simulink library "Environment_Lib"  (Simulink 7.5)
settings: Solver=ode45  SolverMode=SingleTasking  StartTime=0.0  StopTime=10.0  RelTol=1e-3
values from neighbouring files (symbols this model uses):
  Env =     [UAV_modelconfig.mat]
undefined symbols (not defined in the file or in its folder): aeroassertmsg, F, Light, MIL
libraries: simulink x5, aerolibgravity2 x4, Environment_Lib x4, aerolibconvert2 x2, aerolibwind2 x2, aerolibatmos2 x1, aerolibutil x1
settings Model: Creator=Paul Freeman  LastModifiedBy=austinmurch

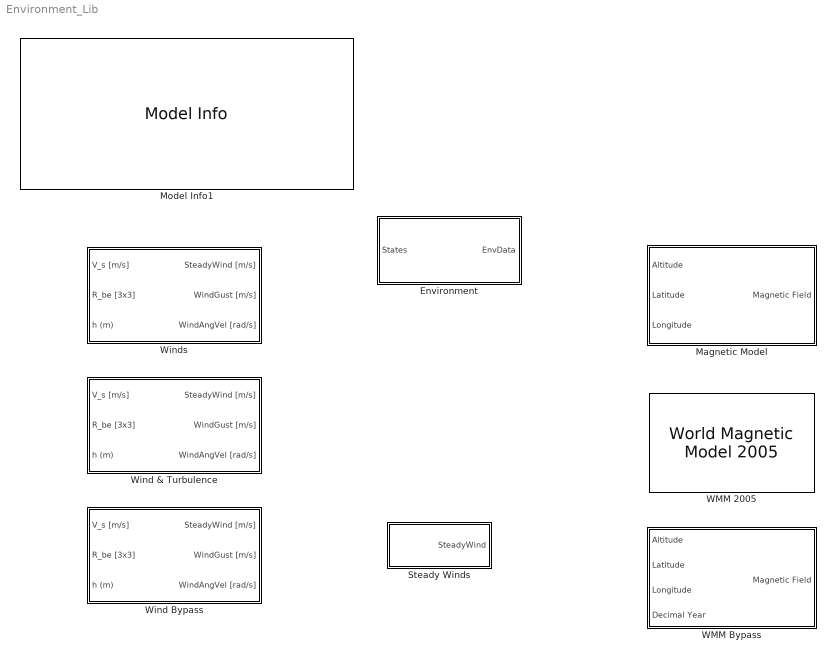
== system Environment_Lib ==
  Environment : Subsystem
  Magnetic Model : Subsystem  BlockChoice=WMM 2005
      settings: TemplateBlock=self  MemberBlocks=WMM 2005,WMM Bypass
  Model Info1 : simulink/Model-Wide Utilities/Model Info  SystemSampleTime=-1  InitialBlockCM=None  BlockCM=None  Frame=on  DisplayStringWithTags=|  HorizontalTextAlignment=Left  LeftAlignmentValue=0.02  SourceBlockDiagram=Environment_Lib  TagMaxNumber=20
      | MODEL INFORMATION
      | Environment Library
      | 
      | University of Minnesota
      | Aerospace Engineering and Mechanics
      | Copyright 2011 Regents of the University of Minnesota. All rights reserved.
      | 
      | == SVN Info ==
      | %<ModelVersion>
      | Last modified by %<LastModifiedBy> on %<LastModificationDate>
  Steady Winds : Subsystem
  WMM 2005 : aerolibgravity2/World Magnetic Model 2005  SystemSampleTime=-1  units=Metric (MKS)  time_in=on  month=August  day=1  year=2009  action=None  h_out=off  dec_out=off  inc_out=off  ti_out=off
  WMM Bypass : Subsystem  AncestorBlock=aerolibgravity2/World Magnetic Model 2005  mask(World Magnetic Model 2005){units=Metric (MKS), time_in=on, month=August, day=1, year=2009, action=None, h_out=off, dec_out=off, inc_out=off, ti_out=off}
      mask prompts: time_in "Input decimal year"; action "Action for out of range input:"; h_out "Output horizontal intensity"; dec_out "Output declination"; inc_out "Output inclination"; ti_out "Output total intensity"
      mask help:
      | Calculate the Earth's magnetic field at a specific location and time using the World Magnetic Model (WMM). This model is valid for the year 2005 through the year 2010.
      |
      | The WMM-2005 can be found on the web at http://www.ngdc.noaa.gov/seg/WMM/DoDWMM.shtml and in "NOAA Technical Report: The US/UK World Magnetic Model for 2005-2010 ".
      |
      | Height is entered in length units of selected unit system. Latitude and longitude are entered in degrees.
      mask init:
      | [ports,dyear,maxdef,epoch,c,cd,fn,fm,snorm,k]=aeroicon('aeroblkwmm2005','icon');
      mask Help: eval('asbhelp');
      mask StyleString: popup(Metric (MKS)|English),checkbox,popup(January|February|March|April|May|June|July|August|September|October|November|December),popup(1|2|3|4|5|6|7|8|9|10|11|12|13|14|15|16|17|18|19|20|21|22|23|24|25|26|27|28|29|30|31),popup(2005|2006|2007|2008|2009|2010),popup(None|Warning|Error),checkbox,checkbox,checkbox,checkbox
      mask CallbackString: |aeroicon('aeroblkwmm');|aeroicon('aeroblkwmm');|aeroicon('aeroblkwmm');|aeroicon('aeroblkwmm');|||||
      mask Display:
      | port_label(ports(1).type,ports(1).port,ports(1).txt);
      | port_label(ports(2).type,ports(2).port,ports(2).txt,'texmode','on');
      | port_label(ports(3).type,ports(3).port,ports(3).txt,'texmode','on');
      | port_label(ports(4).type,ports(4).port,ports(4).txt);
      | port_label(ports(5).type,ports(5).port,ports(5).txt);
      | port_label(ports(6).type,ports(6).port,ports(6).txt);
      | port_label(ports(7).type,ports(7).port,ports(7).txt);
      | port_label(ports(8).type,ports(8).port,ports(8).txt);
      | port_label(ports(9).type,ports(9).port,ports(9).txt);
  Wind & Turbulence : Subsystem
  Wind Bypass : Subsystem
      settings: MinAlgLoopOccurrences=on
  Winds : Subsystem  BlockChoice=Wind & Turbulence
      settings: TemplateBlock=self  MemberBlocks=Wind & Turbulence,Wind Bypass

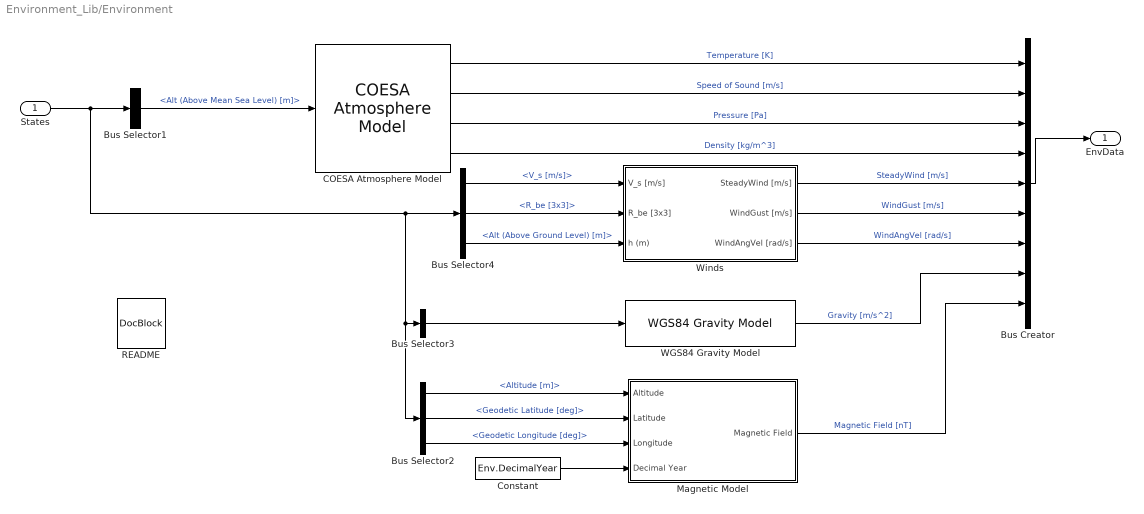
== system Environment_Lib/Environment ==
  States : Inport  OutDataType=sfix(16)  OutScaling=2^0
  Bus Creator : BusCreator  Inputs=9
  Bus Selector1 : BusSelector  OutputSignals=Nav.Alt (Above Mean Sea Level) [m]
  Bus Selector2 : BusSelector  OutputSignals=Nav.Altitude [m],Nav.Geodetic Latitude [deg],Nav.Geodetic Longitude [deg]
  Bus Selector3 : BusSelector  OutputSignals=Nav.Geodetic Latitude [deg],Nav.Geodetic Longitude [deg],Nav.Altitude [m]  OutputAsBus=on
  Bus Selector4 : BusSelector  OutputSignals=WindAxesParam.V_s [m/s],R_be [3x3],Nav.Alt (Above Ground Level) [m]
  COESA Atmosphere Model : aerolibatmos2/COESA Atmosphere Model  SystemSampleTime=-1  units=Metric (MKS)  spec=1976 COESA-extended U.S. Standard Atmosphere  model=Profile  profile_var=High temperature  profile_percent=1%  profile_alt=5 km (16404 ft)  envelope_var=High temperature  envelope_percent=1%  action=Warning
  Constant : Constant  Value=Env.DecimalYear  OutDataType=fixdt(1, 16)  OutScaling=2^0
  Magnetic Model : Subsystem  BlockChoice=WMM 2005
      settings: AttributesFormatString=%<BlockChoice>  TemplateBlock=Environment_Lib/Magnetic Model  MemberBlocks=WMM 2005,WMM Bypass
  README : simulink/Model-Wide Utilities/DocBlock  SystemSampleTime=-1  DocumentType=Text
      content=|
      | Environment Model
      |
      | This block uses the Aerospace Blockset models for Earth's atmosphere,
      | gravity, magnetic field, and wind.
      |
      | The atmosphere is modeled using the 1976 Standard Atmosphere block.
      |
      | Winds are modeled in two portions: steady and unsteady. The steady
      | portion is defined by a speed and direction, and is horizontal only. The
      | unsteady portion is made up of a wind gust model and a turbulence model.
      |
      | The Dryden Wind Turbulence Model is used to model turbulence. The
      | intensity of the turbulence at low altitude (<1000ft) is determined by
      | the wind speed and direction; this is set as separate variables from the
      | steady wind speed and direction. The turbulence is off by default, and
      | can be enabled by setting the Env.Winds.TurbulenceOn boolean in
      | UAV_config.m.
      |
      | The Discrete Gust Model is used to model wind gusts. Parameters are time
      | on, duration (length), and amplitude, in three axes (u,v,w). These
      | parameters are set in Env.Winds, in UAV_config.m
      |
      | Note the booleans in the Env.Winds stucture to turn on each wind
      | component: >> Env.Winds
      |
      | ans =
      |
      |      TurbulenceOn: 0
      |     TurbWindSpeed: 0
      |       TurbWindDir: 0
      |            GustOn: 0
      |     GustStartTime: 0
      |        GustLength: [1 1 1]
      |     GustAmplitude: [1 1 1]
      |      SteadyWindOn: 0
      |         WindSpeed: 0
      |           WindDir: 0
      |
      |
      | The WGS84 Gravity Model is used to model Earth's gravity as a function of
      | latitude, longitude, and altitude.
      |
      | The World Magnetic Model 2005 is used to model Earth's magnetic field as
      | a function of latitude, longitude, and altitude. The current decimal year
      | is input.
      |
      | *Note for trim/linearizing: the Dryden turbulence model and the World
      | Magnetic Model 2005 have many internal states, which makes trimming and
      | linearizing difficult. Thus "Bypass" blocks are substituted for the Winds
      | and Magnetic Model blocks using Configurable Subsystems. For the
      | UAV_NL.mdl, the block choices are automatically set to "Bypass" using the
      | models "InitFcn" callback, which can be viewed by using the Model
      | Explorer, selecting UAV_NL, and going to the "Callbacks" tab. The Nonlinear
      | UAV Model block will then show up as a Parameterized Link (red arrow in the
      | lower left corner). The SIL and PIL sims use the default blocks, and should
      | have a normal library link (black arrow).
  "WGS84 Gravity Model " : aerolibgravity2/WGS84 Gravity Model   SystemSampleTime=-1  model=WGS84 Taylor Series  units=Metric (MKS)  no_atmos=on  precessing=on  jd_loc=off  month=October  day=10  year=2004  no_centrifugal=on  action=Warning
  Winds : Subsystem  BlockChoice=Wind & Turbulence
      settings: AttributesFormatString=%<BlockChoice>  TemplateBlock=Environment_Lib/Winds  MemberBlocks=Wind & Turbulence,Wind Bypass
  EnvData : Outport  OutDataType=sfix(16)  OutScaling=2^0
  wires:
  Bus Selector4/3 -> Winds/3(h (m))  "<Alt (Above Ground Level) [m]>"
  Bus Selector4/2 -> Winds/2(R_be [3x3])  "<R_be [3x3]>"
  Bus Selector4/1 -> Winds/1(V_s [m/s])  "<V_s [m/s]>"
  Bus Creator/1 -> EnvData/1
  Bus Selector1/1 -> COESA Atmosphere Model/1  "<Alt (Above Mean Sea Level) [m]>"
  States/1 -> Bus Selector4/1, Bus Selector3/1, Bus Selector2/1, Bus Selector1/1
  COESA Atmosphere Model/3 -> Bus Creator/3  "Pressure [Pa]"
  COESA Atmosphere Model/2 -> Bus Creator/2  "Speed of Sound [m/s]"
  COESA Atmosphere Model/1 -> Bus Creator/1  "Temperature [K]"
  COESA Atmosphere Model/4 -> Bus Creator/4  "Density [kg/m^3]"
  Winds/1(SteadyWind [m/s]) -> Bus Creator/5  "SteadyWind [m/s]"
  Winds/2(WindGust [m/s]) -> Bus Creator/6  "WindGust [m/s]"
  Winds/3(WindAngVel [rad/s]) -> Bus Creator/7  "WindAngVel [rad/s]"
  "WGS84 Gravity Model "/1 -> Bus Creator/8  "Gravity [m/s^2]"
  Magnetic Model/1(Magnetic Field) -> Bus Creator/9  "Magnetic Field [nT]"
  Bus Selector2/1 -> Magnetic Model/1(Altitude)  "<Altitude [m]>"
  Bus Selector2/2 -> Magnetic Model/2(Latitude)  "<Geodetic Latitude [deg]>"
  Bus Selector2/3 -> Magnetic Model/3(Longitude)  "<Geodetic Longitude [deg]>"
  Bus Selector3/1 -> "WGS84 Gravity Model "/1
  Constant/1 -> Magnetic Model/4(Decimal Year)

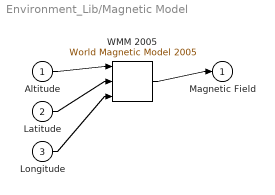
== system Environment_Lib/Magnetic Model ==
  Altitude : Inport
  Latitude : Inport  Port=2
  Longitude : Inport  Port=3
  WMM 2005 : aerolibgravity2/World Magnetic Model 2005  SystemSampleTime=-1  units=Metric (MKS)  time_in=off  month=August  day=1  year=2009  action=None  h_out=off  dec_out=off  inc_out=off  ti_out=off
  Magnetic Field : Outport
  wires:
  Altitude/1 -> WMM 2005/1
  Latitude/1 -> WMM 2005/2
  Longitude/1 -> WMM 2005/3
  WMM 2005/1 -> Magnetic Field/1

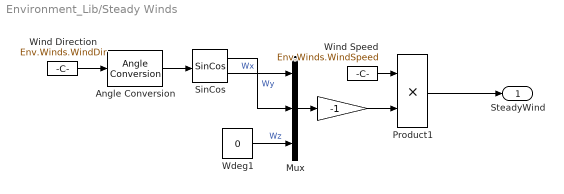
== system Environment_Lib/Steady Winds ==
  " " : Gain  Gain=-1  ParameterDataType=sfix(16)  ParameterScaling=2^0  OutDataType=sfix(16)  OutScaling=2^0  SaturateOnIntegerOverflow=on  OutDataTypeStr=Inherit: Same as input  ParamDataTypeStr=Inherit: Same as input
  Angle Conversion : aerolibconvert2/Angle Conversion  SystemSampleTime=-1  IU=deg  OU=rad
  Mux : Mux  Inputs=3
  Product1 : Product  OutDataType=sfix(16)  OutScaling=2^0  SaturateOnIntegerOverflow=on  InputSameDT=on  OutDataTypeStr=Inherit: Same as first input
  SinCos : aerolibutil/SinCos  SystemSampleTime=-1
  Wdeg1 : Constant  Value=0  OutDataType=sfix(16)  OutScaling=2^0  OutDataTypeStr=Inherit: Inherit via back propagation
  Wind Direction : Constant  Value=Env.Winds.WindDir  OutDataType=sfix(16)  OutScaling=2^0  OutDataTypeStr=Inherit: Inherit via back propagation
  Wind Speed : Constant  Value=Env.Winds.WindSpeed  OutDataType=sfix(16)  OutScaling=2^0  OutDataTypeStr=Inherit: Inherit via back propagation
  SteadyWind : Outport  OutDataType=fixdt(1, 16)  OutScaling=2^0
  wires:
  " "/1 -> Product1/2
  Product1/1 -> SteadyWind/1
  Mux/1 -> " "/1
  Wdeg1/1 -> Mux/3  "Wz"
  Angle Conversion/1 -> SinCos/1
  SinCos/1 -> Mux/2  "Wy"
  SinCos/2 -> Mux/1  "Wx"
  Wind Speed/1 -> Product1/1
  Wind Direction/1 -> Angle Conversion/1

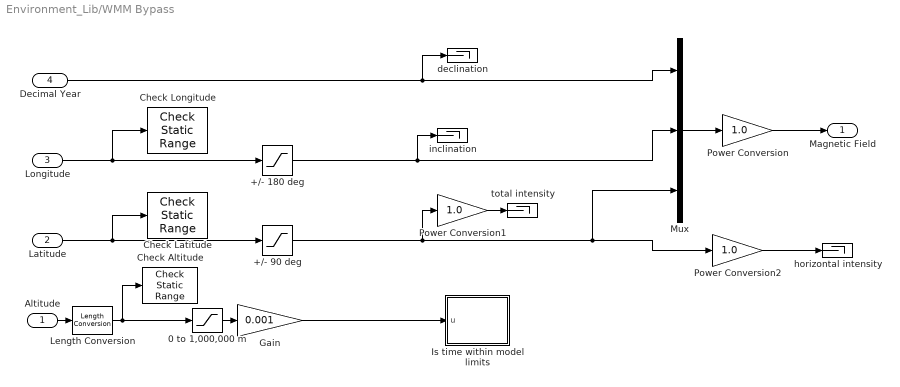
== system Environment_Lib/WMM Bypass ==
  Altitude : Inport  OutDataType=sfix(16)  OutScaling=2^0
  Latitude : Inport  Port=2  OutDataType=sfix(16)  OutScaling=2^0
  Longitude : Inport  Port=3  OutDataType=sfix(16)  OutScaling=2^0
  Decimal Year : Inport  Port=4
  +/- 180 deg : Saturate  UpperLimit=180.0  LowerLimit=-180.0  OutDataType=sfix(16)  OutScaling=2^0
  +/- 90 deg : Saturate  UpperLimit=90.0  LowerLimit=-90.0  OutDataType=sfix(16)  OutScaling=2^0
  0 to 1,000,000 m : Saturate  UpperLimit=1000000.0  LowerLimit=0  OutDataType=sfix(16)  OutScaling=2^0
  Check Altitude : simulink/Model Verification/Check  Static Range  Description=0 <= u <= 1000000  SystemSampleTime=-1  max=1000000  max_included=on  min=0  min_included=on  enabled=off  callback=aeroassertmsg('aeroblkwmm','alt');  stopWhenAssertionFail=off  export=off  icon=graphic
  Check Latitude : simulink/Model Verification/Check  Static Range  Description=-90 <= u <= 90  SystemSampleTime=-1  max=90  max_included=on  min=-90  min_included=on  enabled=off  callback=aeroassertmsg('aeroblkwmm','lat');  stopWhenAssertionFail=off  export=off  icon=graphic
  Check Longitude : simulink/Model Verification/Check  Static Range  Description=-180 <= u <= 180  SystemSampleTime=-1  max=180  max_included=on  min=-180  min_included=on  enabled=off  callback=aeroassertmsg('aeroblkwmm','lon');  stopWhenAssertionFail=off  export=off  icon=graphic
  Gain : Gain  Gain=0.001  ParameterDataType=sfix(16)  ParameterScaling=2^0  OutDataType=sfix(16)  OutScaling=2^0  SaturateOnIntegerOverflow=on  OutDataTypeStr=Inherit: Same as input  ParamDataTypeStr=Inherit: Same as input
  Is time within model limits : Subsystem  Description=0 <= u <= 5  mask(Checks_SRange){max=5, max_included=on, min=0, min_included=on, enabled=off, callback=aeroassertmsg('aeroblkwmm','time');, stopWhenAssertionFail=off, export=off, icon=graphic}
      mask prompts: max "Upper bound:"; max_included "Inclusive upper bound"; min "Lower bound:"; min_included "Inclusive lower bound"; enabled "Enable assertion"; callback "Simulation callback when assertion fails (optional):"; stopWhenAssertionFail "Stop simulation when assertion fails"; export "Output assertion signal"; icon "Select icon type:"
      mask help: Assert that the input signal lies between a static lower and upper bound or optionally equals either bound.
      mask init:
      | update_assert_sys(gcbh);
      mask StyleString: edit,checkbox,edit,checkbox,checkbox,edit,checkbox,checkbox,popup(graphic|text)
      mask Display:
      | image(imread('Checks_SRange.bmp','bmp'),'center')
      | plot([0 1], [0 1]);
      | plot([0 1],[1 0]);
  Length Conversion : aerolibconvert2/Length Conversion  SystemSampleTime=-1  IU=m  OU=m
  Mux : Mux  Inputs=3
  Power Conversion : Gain  Gain=1.0  ParameterDataType=sfix(16)  ParameterScaling=2^0  OutDataType=sfix(16)  OutScaling=2^0  SaturateOnIntegerOverflow=on  OutDataTypeStr=Inherit: Same as input  ParamDataTypeStr=Inherit: Same as input
  Power Conversion1 : Gain  Gain=1.0  ParameterDataType=sfix(16)  ParameterScaling=2^0  OutDataType=sfix(16)  OutScaling=2^0  SaturateOnIntegerOverflow=on  OutDataTypeStr=Inherit: Same as input  ParamDataTypeStr=Inherit: Same as input
  Power Conversion2 : Gain  Gain=1.0  ParameterDataType=sfix(16)  ParameterScaling=2^0  OutDataType=sfix(16)  OutScaling=2^0  SaturateOnIntegerOverflow=on  OutDataTypeStr=Inherit: Same as input  ParamDataTypeStr=Inherit: Same as input
  declination : Terminator
  horizontal intensity : Terminator
  inclination : Terminator
  total intensity : Terminator
  Magnetic Field : Outport  OutDataType=sfix(16)  OutScaling=2^0
  wires:
  Altitude/1 -> Length Conversion/1
  Length Conversion/1 -> 0 to 1,000,000 m/1, Check Altitude/1
  Decimal Year/1 -> declination/1, Mux/1
  Latitude/1 -> +/- 90 deg/1, Check Latitude/1
  Longitude/1 -> +/- 180 deg/1, Check Longitude/1
  Gain/1 -> Is time within model limits/1(u)
  Mux/1 -> Power Conversion/1
  Power Conversion/1 -> Magnetic Field/1
  Power Conversion1/1 -> total intensity/1
  Power Conversion2/1 -> horizontal intensity/1
  +/- 90 deg/1 -> Power Conversion1/1, Power Conversion2/1, Mux/3
  +/- 180 deg/1 -> inclination/1, Mux/2
  0 to 1,000,000 m/1 -> Gain/1

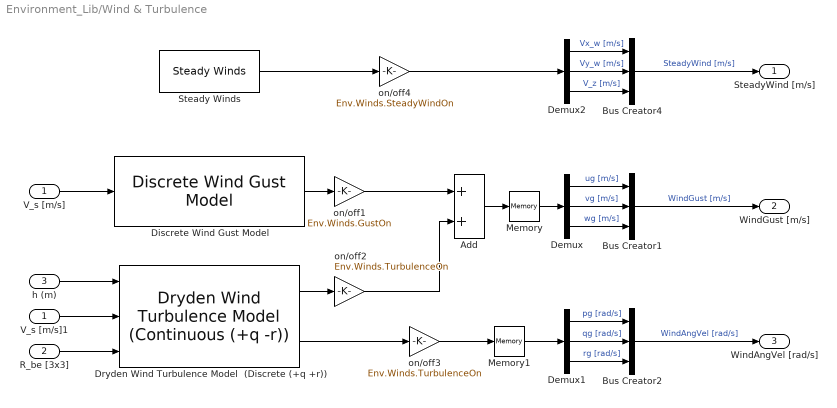
== system Environment_Lib/Wind & Turbulence ==
  V_s [m/s] : Inport  OutDataType=sfix(16)  OutScaling=2^0
  R_be [3x3] : Inport  Port=2  OutDataType=sfix(16)  OutScaling=2^0
  h (m) : Inport  Port=3  OutDataType=sfix(16)  OutScaling=2^0
  Add : Sum  OutDataType=fixdt(1, 16)  OutScaling=2^-10
  Bus Creator1 : BusCreator  Inputs=3
  Bus Creator2 : BusCreator  Inputs=3
  Bus Creator4 : BusCreator  Inputs=3
  Demux : Demux  Outputs=3
  Demux1 : Demux  Outputs=3
  Demux2 : Demux  Outputs=3
  Discrete Wind Gust Model : aerolibwind2/Discrete Wind Gust Model  SystemSampleTime=-1  units=Metric (MKS)  Gx=on  Gy=on  Gz=on  t_0=Env.Winds.GustStartTime  d_m=Env.Winds.GustLength  v_m=Env.Winds.GustAmplitude
  Dryden Wind Turbulence Model  (Discrete (+q +r)) : aerolibwind2/Dryden Wind Turbulence Model  (Continuous (+q -r))  SystemSampleTime=-1  units=Metric (MKS)  spec=MIL-F-8785C  model=Discrete Dryden (+q +r)  W20=Env.Winds.TurbWindSpeed  Wdeg=Env.Winds.TurbWindDir  TurbProb=10^-2 - Light  L_high=762  Wingspan=AC.Geometry.b  ts=SampleTime  Seed=[23341 23342 23343 23344]  T_on=on
  Memory : Memory
  Memory1 : Memory
  Steady Winds : Environment_Lib/Steady Winds  SystemSampleTime=-1
  V_s [m/s]1 : InportShadow  Port=1  OutDataType=sfix(16)  OutScaling=2^0
  on/off1 : Gain  Gain=Env.Winds.GustOn  ParameterDataType=fixdt(1, 16)  ParameterScaling=2^0  OutDataType=fixdt(1, 16)  OutScaling=2^0
  on/off2 : Gain  Gain=Env.Winds.TurbulenceOn  ParameterDataType=fixdt(1, 16)  ParameterScaling=2^0  OutDataType=fixdt(1, 16)  OutScaling=2^0
  on/off3 : Gain  Gain=Env.Winds.TurbulenceOn  ParameterDataType=fixdt(1, 16)  ParameterScaling=2^0  OutDataType=fixdt(1, 16)  OutScaling=2^0
  on/off4 : Gain  Gain=Env.Winds.SteadyWindOn  ParameterDataType=fixdt(1, 16)  ParameterScaling=2^0  OutDataType=fixdt(1, 16)  OutScaling=2^0
  SteadyWind [m/s] : Outport  OutDataType=sfix(16)  OutScaling=2^0
  WindGust [m/s] : Outport  Port=2  OutDataType=sfix(16)  OutScaling=2^0
  WindAngVel [rad/s] : Outport  Port=3  OutDataType=sfix(16)  OutScaling=2^0
  wires:
  Demux/1 -> Bus Creator1/1  "ug [m/s]"
  Demux1/3 -> Bus Creator2/3  "rg [rad/s]"
  Demux1/2 -> Bus Creator2/2  "qg [rad/s]"
  Demux1/1 -> Bus Creator2/1  "pg [rad/s]"
  Demux/3 -> Bus Creator1/3  "wg [m/s]"
  Demux/2 -> Bus Creator1/2  "vg [m/s]"
  V_s [m/s]/1 -> Discrete Wind Gust Model/1
  Demux2/1 -> Bus Creator4/1  "Vx_w [m/s]"
  Demux2/3 -> Bus Creator4/3  "V_z [m/s]"
  Demux2/2 -> Bus Creator4/2  "Vy_w [m/s]"
  Steady Winds/1 -> on/off4/1
  Add/1 -> Memory/1
  Discrete Wind Gust Model/1 -> on/off1/1
  Dryden Wind Turbulence Model  (Discrete (+q +r))/1 -> on/off2/1
  on/off3/1 -> Memory1/1
  on/off4/1 -> Demux2/1
  on/off1/1 -> Add/1
  on/off2/1 -> Add/2
  Memory/1 -> Demux/1
  Memory1/1 -> Demux1/1
  Bus Creator4/1 -> SteadyWind [m/s]/1  "SteadyWind [m/s]"
  Bus Creator1/1 -> WindGust [m/s]/1  "WindGust [m/s]"
  Bus Creator2/1 -> WindAngVel [rad/s]/1  "WindAngVel [rad/s]"
  Dryden Wind Turbulence Model  (Discrete (+q +r))/2 -> on/off3/1
  R_be [3x3]/1 -> Dryden Wind Turbulence Model  (Discrete (+q +r))/3
  h (m)/1 -> Dryden Wind Turbulence Model  (Discrete (+q +r))/1
  V_s [m/s]1/1 -> Dryden Wind Turbulence Model  (Discrete (+q +r))/2

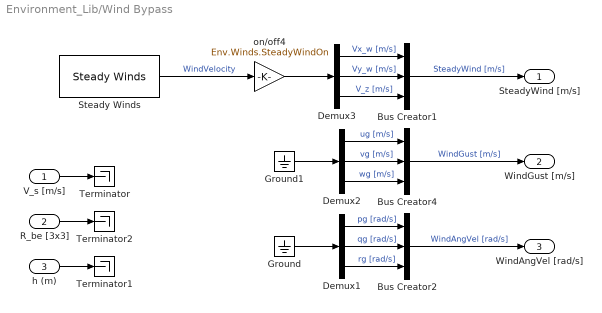
== system Environment_Lib/Wind Bypass ==
  V_s [m/s] : Inport  OutDataType=sfix(16)  OutScaling=2^0
  R_be [3x3] : Inport  Port=2  OutDataType=sfix(16)  OutScaling=2^0
  h (m) : Inport  Port=3  OutDataType=sfix(16)  OutScaling=2^0
  Bus Creator1 : BusCreator  Inputs=3
  Bus Creator2 : BusCreator  Inputs=3
  Bus Creator4 : BusCreator  Inputs=3
  Demux1 : Demux  Outputs=3
  Demux2 : Demux  Outputs=3
  Demux3 : Demux  Outputs=3
  Ground : Ground
  Ground1 : Ground
  Steady Winds : Environment_Lib/Steady Winds  SystemSampleTime=-1
  Terminator : Terminator
  Terminator1 : Terminator
  Terminator2 : Terminator
  on/off4 : Gain  Gain=Env.Winds.SteadyWindOn  ParameterDataType=fixdt(1, 16)  ParameterScaling=2^0  OutDataType=fixdt(1, 16)  OutScaling=2^0
  SteadyWind [m/s] : Outport  OutDataType=sfix(16)  OutScaling=2^0
  WindGust [m/s] : Outport  Port=2  OutDataType=sfix(16)  OutScaling=2^0
  WindAngVel [rad/s] : Outport  Port=3  OutDataType=sfix(16)  OutScaling=2^0
  wires:
  Demux1/3 -> Bus Creator2/3  "rg [rad/s]"
  Demux1/2 -> Bus Creator2/2  "qg [rad/s]"
  Demux1/1 -> Bus Creator2/1  "pg [rad/s]"
  Steady Winds/1 -> on/off4/1  "WindVelocity"
  V_s [m/s]/1 -> Terminator/1
  Ground/1 -> Demux1/1
  Demux2/1 -> Bus Creator4/1  "ug [m/s]"
  Demux2/3 -> Bus Creator4/3  "wg [m/s]"
  Demux2/2 -> Bus Creator4/2  "vg [m/s]"
  Ground1/1 -> Demux2/1
  Demux3/1 -> Bus Creator1/1  "Vx_w [m/s]"
  Demux3/3 -> Bus Creator1/3  "V_z [m/s]"
  Demux3/2 -> Bus Creator1/2  "Vy_w [m/s]"
  on/off4/1 -> Demux3/1
  Bus Creator1/1 -> SteadyWind [m/s]/1  "SteadyWind [m/s]"
  Bus Creator4/1 -> WindGust [m/s]/1  "WindGust [m/s]"
  Bus Creator2/1 -> WindAngVel [rad/s]/1  "WindAngVel [rad/s]"
  R_be [3x3]/1 -> Terminator2/1
  h (m)/1 -> Terminator1/1

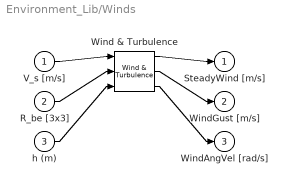
== system Environment_Lib/Winds ==
  V_s [m/s] : Inport
  R_be [3x3] : Inport  Port=2
  h (m) : Inport  Port=3
  Wind & Turbulence : Environment_Lib/Wind & Turbulence  SystemSampleTime=-1
  SteadyWind [m/s] : Outport
  WindGust [m/s] : Outport  Port=2
  WindAngVel [rad/s] : Outport  Port=3
  wires:
  V_s [m/s]/1 -> Wind & Turbulence/1
  R_be [3x3]/1 -> Wind & Turbulence/2
  h (m)/1 -> Wind & Turbulence/3
  Wind & Turbulence/1 -> SteadyWind [m/s]/1
  Wind & Turbulence/2 -> WindGust [m/s]/1
  Wind & Turbulence/3 -> WindAngVel [rad/s]/1

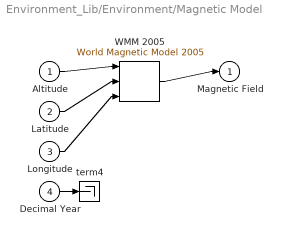
== system Environment_Lib/Environment/Magnetic Model ==
  Altitude : Inport
  Latitude : Inport  Port=2
  Longitude : Inport  Port=3
  Decimal Year : Inport  Port=4
  WMM 2005 : aerolibgravity2/World Magnetic Model 2005  SystemSampleTime=-1  units=Metric (MKS)  time_in=off  month=August  day=1  year=2009  action=None  h_out=off  dec_out=off  inc_out=off  ti_out=off
  term4 : Terminator
  Magnetic Field : Outport
  wires:
  Altitude/1 -> WMM 2005/1
  Latitude/1 -> WMM 2005/2
  Longitude/1 -> WMM 2005/3
  WMM 2005/1 -> Magnetic Field/1
  Decimal Year/1 -> term4/1

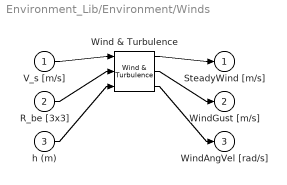
== system Environment_Lib/Environment/Winds ==
  V_s [m/s] : Inport
  R_be [3x3] : Inport  Port=2
  h (m) : Inport  Port=3
  Wind & Turbulence : Environment_Lib/Wind & Turbulence  SystemSampleTime=-1
  SteadyWind [m/s] : Outport
  WindGust [m/s] : Outport  Port=2
  WindAngVel [rad/s] : Outport  Port=3
  wires:
  V_s [m/s]/1 -> Wind & Turbulence/1
  R_be [3x3]/1 -> Wind & Turbulence/2
  h (m)/1 -> Wind & Turbulence/3
  Wind & Turbulence/1 -> SteadyWind [m/s]/1
  Wind & Turbulence/2 -> WindGust [m/s]/1
  Wind & Turbulence/3 -> WindAngVel [rad/s]/1

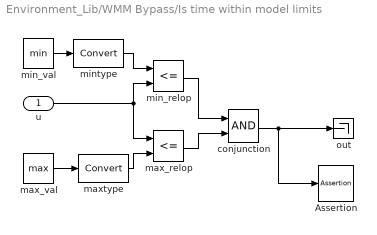
== system Environment_Lib/WMM Bypass/Is time within model limits ==
  u : Inport  OutDataType=sfix(16)  OutScaling=2^0
  Assertion : Assertion  Enabled=off  AssertionFailFcn=aeroassertmsg('aeroblkwmm','time');  StopWhenAssertionFail=off
  conjunction : Logic
  max_relop : RelationalOperator  Operator=<=  InputSameDT=on
  max_val : Constant  Value=max  OutDataType=sfix(16)  OutScaling=2^0
  maxtype : DataTypeConversion  OutDataType=sfix(16)  OutScaling=2^0  SaturateOnIntegerOverflow=on  RndMeth=Zero
  min_relop : RelationalOperator  Operator=<=  InputSameDT=on
  min_val : Constant  Value=min  OutDataType=sfix(16)  OutScaling=2^0
  mintype : DataTypeConversion  OutDataType=sfix(16)  OutScaling=2^0  SaturateOnIntegerOverflow=on  RndMeth=Zero
  out : Terminator
  wires:
  maxtype/1 -> max_relop/2
  mintype/1 -> min_relop/1
  conjunction/1 -> Assertion/1, out/1
  max_relop/1 -> conjunction/2
  min_relop/1 -> conjunction/1
  max_val/1 -> maxtype/1
  min_val/1 -> mintype/1
  u/1 -> max_relop/1, min_relop/2
